simulink model "base_1fm"  (R2016b)
settings: Solver=VariableStepAuto  StartTime=0.0  StopTime=10.0  RelTol=1e-3
values from neighbouring files (symbols this model uses):
  Lb = 0.07    [base_1fm_parameters.m]
  Lf = 0.238    [base_1fm_parameters.m]
  Lu = 0.153    [base_1fm_parameters.m]
  sampleTime = 0.001    [base_1fm_parameters.m]
undefined symbols (not defined in the file or in its folder): DiscIntNeverNeededParam, RobotStruct
undefined symbols (not defined in the file): RobotStruct_FM1
libraries: simulink x27, VariousBlocksLibrary x4, FMLibrary_v2 x2, UsefulBlocksLibrary x2, simulink_extras x2, FM_Library x1
(part 2 of 3)

== system base_1fm/Robot1/DataToEtherCAT/ToActuator ==
  note: The Latched version keeps the most recent value from when the motor was on; in other words, the reason why the motor turned off.
  note: The UseActuator block can be used to enable or disable the actuator altogether.
  BusActuator : Inport
  DriveErrorIn : Inport  Port=2
  WorkspaceErrorIn : Inport  Port=3
  EnableDrive : Inport  Port=4
  DisableDrive : Inport  Port=5
  JointTorqueDes_rad : Inport  Port=6
  AppendToBus : Subsystem
  DriveEnableLogic : Subsystem
  EncodeDesiredTorque : MATLAB Function  TreatAsAtomicUnit=on  mask(EncodeDesiredTorque){transmissionRatio=ActuatorStruct.transmissionRatio, motorTorqueConstant=ActuatorStruct.motorTorqueConstant, drivePeakCurrent=ActuatorStruct.drivePeakCurrent}
      mask prompts: transmissionRatio "Transmission ratio (e.g. -8) [-]"; motorTorqueConstant "Motor torque constant [Nm/A]"; drivePeakCurrent "Motor drive peak current [A]"
      mask help:
      | Encode desired torque at the joint to torque to be produced by the motor.
      |
      | Note: due to the way the transmission is set up and the positive motor axis (clockwise is positive as seen from the motor front), there is no need to account for sign change in motor torque or encoder position.
  PreventAlgebraicLoop : Memory
  TorqueLimit_Nm : Constant  Value=ActuatorStruct.TorqueLimit_Nm
  TorqueLimiter : FM_Library/TorqueLimiter
  UseActuator : Constant  OutDataTypeStr=double
      settings: OpenFcn=|
      | b = get_param(gcb,'value');
      | if (strcmp(b,'1')),
      |   set_param (gcb,'value','0');
      | else
      |   set_param(gcb,'value','1');
      | end;
  Enable_enablecircuit : Outport
  ControlWord_drive : Outport  Port=2
  ModesOfOperation_drive : Outport  Port=3
  TargetCurrent_Drive : Outport  Port=4
  DriveErrorOut : Outport  Port=5
  DriveErrorLatched : Outport  Port=6
  ToLogger : Outport  Port=7
  wires:
  WorkspaceErrorIn/1 -> DriveEnableLogic/5(WorkspaceErrorIn)
  DriveEnableLogic/1(Enable_enablecircuit) -> Enable_enablecircuit/1
  JointTorqueDes_rad/1 -> AppendToBus/3(DesiredTorque), TorqueLimiter/2
  TorqueLimiter/1 -> DriveEnableLogic/7(TorqueGuardMax)
  TorqueLimiter/2 -> AppendToBus/4(DesiredTorqueLimited), EncodeDesiredTorque/1(JointTorque_Des_Nm)
  DriveEnableLogic/5(DriveErrorOutLatched) -> DriveErrorLatched/1
  TorqueLimit_Nm/1 -> TorqueLimiter/1
  DriveEnableLogic/3(ModesOfOperation_drive) -> ModesOfOperation_drive/1
  DriveEnableLogic/2(ControlWord_drive) -> ControlWord_drive/1
  EncodeDesiredTorque/1(MotorTorque_Des_IU) -> TargetCurrent_Drive/1
  BusActuator/1 -> DriveEnableLogic/6(BusActuators), AppendToBus/1(Bus_in)
  EnableDrive/1 -> DriveEnableLogic/1(EnableDrive)
  DisableDrive/1 -> DriveEnableLogic/2(DisableDrive)
  DriveEnableLogic/4(DriveErrorOut) -> AppendToBus/2(DriveError), PreventAlgebraicLoop/1
  DriveErrorIn/1 -> DriveEnableLogic/4(DriveErrorIn)
  PreventAlgebraicLoop/1 -> DriveErrorOut/1
  AppendToBus/1(Bus_out) -> ToLogger/1
  UseActuator/1 -> DriveEnableLogic/3(UseActuator)

== system base_1fm/Robot1/DataToEtherCAT/ToActuator1 ==
  note: The Latched version keeps the most recent value from when the motor was on; in other words, the reason why the motor turned off.
  note: The UseActuator block can be used to enable or disable the actuator altogether.
  BusActuator : Inport
  DriveErrorIn : Inport  Port=2
  WorkspaceErrorIn : Inport  Port=3
  EnableDrive : Inport  Port=4
  DisableDrive : Inport  Port=5
  JointTorqueDes_rad : Inport  Port=6
  AppendToBus : Subsystem
  DriveEnableLogic : Subsystem
  EncodeDesiredTorque : MATLAB Function  TreatAsAtomicUnit=on  mask(EncodeDesiredTorque){transmissionRatio=ActuatorStruct.transmissionRatio, motorTorqueConstant=ActuatorStruct.motorTorqueConstant, drivePeakCurrent=ActuatorStruct.drivePeakCurrent}
      mask prompts: transmissionRatio "Transmission ratio (e.g. -8) [-]"; motorTorqueConstant "Motor torque constant [Nm/A]"; drivePeakCurrent "Motor drive peak current [A]"
      mask help:
      | Encode desired torque at the joint to torque to be produced by the motor.
      |
      | Note: due to the way the transmission is set up and the positive motor axis (clockwise is positive as seen from the motor front), there is no need to account for sign change in motor torque or encoder position.
  PreventAlgebraicLoop : Memory
  TorqueLimit_Nm : Constant  Value=ActuatorStruct.TorqueLimit_Nm
  TorqueLimiter1 : Subsystem  AncestorBlock=FMLibrary_v2/Utilities/TorqueLimiter
  UseActuator : Constant  OutDataTypeStr=double
      settings: OpenFcn=|
      | b = get_param(gcb,'value');
      | if (strcmp(b,'1')),
      |   set_param (gcb,'value','0');
      | else
      |   set_param(gcb,'value','1');
      | end;
  Enable_enablecircuit : Outport
  ControlWord_drive : Outport  Port=2
  ModesOfOperation_drive : Outport  Port=3
  TargetCurrent_Drive : Outport  Port=4
  DriveErrorOut : Outport  Port=5
  DriveErrorLatched : Outport  Port=6
  ToLogger : Outport  Port=7
  wires:
  WorkspaceErrorIn/1 -> DriveEnableLogic/5(WorkspaceErrorIn)
  DriveEnableLogic/1(Enable_enablecircuit) -> Enable_enablecircuit/1
  JointTorqueDes_rad/1 -> TorqueLimiter1/2(Torque_Des_Nm), AppendToBus/3(DesiredTorque)
  TorqueLimiter1/1(Torque_GuardMax_Nm) -> DriveEnableLogic/7(TorqueGuardMax)
  TorqueLimiter1/2(Torque_Des_Limited_Nm) -> AppendToBus/4(DesiredTorqueLimited), EncodeDesiredTorque/1(JointTorque_Des_Nm)
  DriveEnableLogic/5(DriveErrorOutLatched) -> DriveErrorLatched/1
  TorqueLimit_Nm/1 -> TorqueLimiter1/1(Torque_Limit_Nm)
  DriveEnableLogic/3(ModesOfOperation_drive) -> ModesOfOperation_drive/1
  DriveEnableLogic/2(ControlWord_drive) -> ControlWord_drive/1
  EncodeDesiredTorque/1(MotorTorque_Des_IU) -> TargetCurrent_Drive/1
  BusActuator/1 -> DriveEnableLogic/6(BusActuators), AppendToBus/1(Bus_in)
  EnableDrive/1 -> DriveEnableLogic/1(EnableDrive)
  DisableDrive/1 -> DriveEnableLogic/2(DisableDrive)
  DriveEnableLogic/4(DriveErrorOut) -> AppendToBus/2(DriveError), PreventAlgebraicLoop/1
  DriveErrorIn/1 -> DriveEnableLogic/4(DriveErrorIn)
  PreventAlgebraicLoop/1 -> DriveErrorOut/1
  AppendToBus/1(Bus_out) -> ToLogger/1
  UseActuator/1 -> DriveEnableLogic/3(UseActuator)

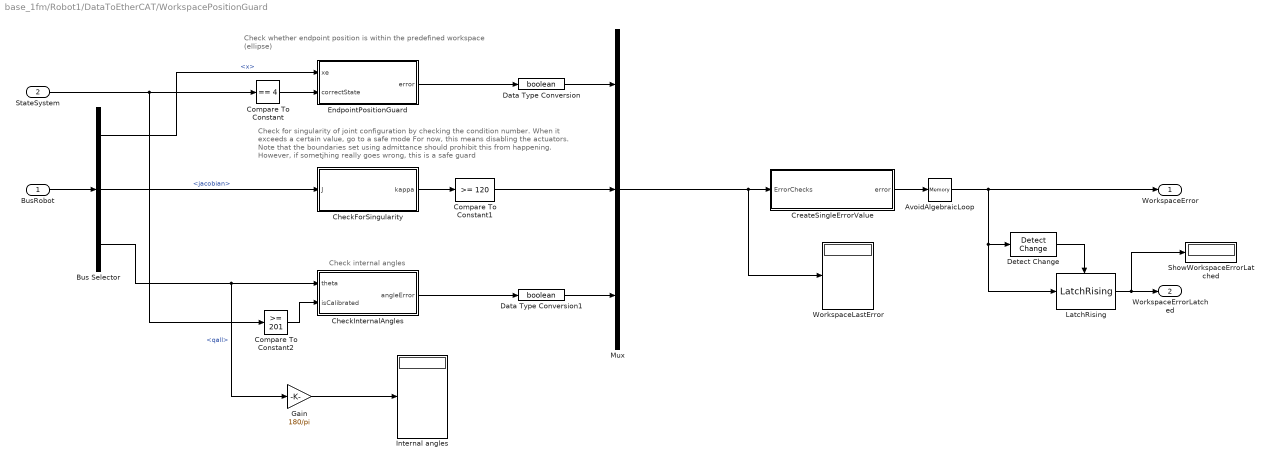
== system base_1fm/Robot1/DataToEtherCAT/WorkspacePositionGuard ==
  note: Check for singularity of joint configuration by checking
      | the condition number. When it exceeds a certain value, go to a safe mode
      | For now, this means disabling the actuators.
      | Note that the boundaries set using admittance should prohibit this from happening.
      | However, if sometjhing really goes wrong, this is a safe guard
  note: Check whether endpoint position is within the predefined workspace
      | (ellipse)
  note: Check internal angles
  BusRobot : Inport
  StateSystem : Inport  Port=2
  AvoidAlgebraicLoop : Memory
  Bus Selector : BusSelector  OutputSignals=xOpSpace.x,xOpSpace.jacobian,qJointSpace.qall
  CheckForSingularity : MATLAB Function  TreatAsAtomicUnit=on
  CheckInternalAngles : MATLAB Function  TreatAsAtomicUnit=on
  Compare To Constant : simulink/Logic and Bit Operations/Compare To Constant  relop===  const=4  OutDataTypeStr=boolean
  Compare To Constant1 : simulink/Logic and Bit Operations/Compare To Constant  relop=>=  const=120  OutDataTypeStr=boolean
  Compare To Constant2 : simulink/Logic and Bit Operations/Compare To Constant  relop=>=  const=201  OutDataTypeStr=boolean
  CreateSingleErrorValue : Subsystem
  Data Type Conversion : DataTypeConversion  OutDataTypeStr=boolean
  Data Type Conversion1 : DataTypeConversion  OutDataTypeStr=boolean
  Detect Change : simulink/Logic and Bit Operations/Detect Change  vinit=0  InputProcessing=Inherited  OutDataTypeStr=boolean
  EndpointPositionGuard : MATLAB Function  TreatAsAtomicUnit=on
  Gain : Gain  Gain=180/pi
  Internal angles : Display
  LatchRising : UsefulBlocksLibrary/LatchRising  ic=0
  Mux : Mux  Inputs=3
  ShowWorkspaceErrorLatched : Display
  WorkspaceLastError : Display
  WorkspaceError : Outport
  WorkspaceErrorLatched : Outport  Port=2
  wires:
  StateSystem/1 -> Compare To Constant/1, Compare To Constant2/1
  Bus Selector/2 -> CheckForSingularity/1(J)  "<jacobian>"
  Gain/1 -> Internal angles/1
  Compare To Constant2/1 -> CheckInternalAngles/2(isCalibrated)
  Compare To Constant/1 -> EndpointPositionGuard/2(correctState)
  AvoidAlgebraicLoop/1 -> WorkspaceError/1, LatchRising/1, Detect Change/1
  Detect Change/1 -> LatchRising/Trigger
  CreateSingleErrorValue/1(error) -> AvoidAlgebraicLoop/1
  Data Type Conversion1/1 -> Mux/3
  Data Type Conversion/1 -> Mux/1
  Compare To Constant1/1 -> Mux/2
  LatchRising/1 -> WorkspaceErrorLatched/1, ShowWorkspaceErrorLatched/1
  CheckInternalAngles/1(angleError) -> Data Type Conversion1/1
  Bus Selector/3 -> CheckInternalAngles/1(theta), Gain/1  "<qall>"
  Bus Selector/1 -> EndpointPositionGuard/1(xe)  "<x>"
  BusRobot/1 -> Bus Selector/1
  EndpointPositionGuard/1(error) -> Data Type Conversion/1
  Mux/1 -> CreateSingleErrorValue/1(ErrorChecks), WorkspaceLastError/1
  CheckForSingularity/1(kappa) -> Compare To Constant1/1

== system base_1fm/Robot1/Controller/PD + Nonlinear ID/AFFC ==
  q_ref : Inport
  qdot_ref : Inport  Port=2
  qddot_ref : Inport  Port=3
  e : Inport  Port=4
  Enable : EnablePort  StatesWhenEnabling=reset
  AFFC : MATLAB Function  TreatAsAtomicUnit=on
  Counter Free-Running : simulink/Sources/Counter Free-Running  NumBits=32  tsamp=-1
  Data Type Conversion : DataTypeConversion  OutDataTypeStr=double
  Learning factors : Constant  Value=[2e-5;1e-2;1e-3;1e-3]
  sample time : Gain  Gain=sampleTime
  p : Outport  OutputWhenDisabled=reset
  tau_affc : Outport  Port=2  OutputWhenDisabled=reset  InitialOutput=[0;0]
  wires:
  Learning factors/1 -> AFFC/6(w)
  Data Type Conversion/1 -> sample time/1
  sample time/1 -> AFFC/1(t)
  Counter Free-Running/1 -> Data Type Conversion/1
  AFFC/1(p) -> p/1
  AFFC/2(tau) -> tau_affc/1
  q_ref/1 -> AFFC/2(q)
  qdot_ref/1 -> AFFC/3(qdot)
  qddot_ref/1 -> AFFC/4(qddot)
  e/1 -> AFFC/5(e)

== system base_1fm/Robot1/DataFromEtherCAT/Calculate Arrange Joint and Op Space/forward kinematics ==
  JointPosition_rad : Inport  PortDimensions=[2 1]
  JointVelocity_rads : Inport  Port=2  PortDimensions=[2 1]
  JointAcceleration_rads2 : Inport  Port=3  PortDimensions=[2 1]
  Je : MATLAB Function  TreatAsAtomicUnit=on
  Jedot : MATLAB Function  TreatAsAtomicUnit=on
  Product : Product  Multiplication=Matrix(*)
  calculate xddot : MATLAB Function  TreatAsAtomicUnit=on
  forward kinematics : MATLAB Function  TreatAsAtomicUnit=on
  x : Outport
  xdot : Outport  Port=2
  xddot : Outport  Port=3
  J : Outport  Port=4
  Jdot : Outport  Port=5
  wires:
  JointAcceleration_rads2/1 -> calculate xddot/1(qddot)
  calculate xddot/1(xddot) -> xddot/1
  forward kinematics/1(x) -> x/1
  Product/1 -> xdot/1
  Jedot/1(Jedot) -> Jdot/1, calculate xddot/4(Jdot)
  JointVelocity_rads/1 -> Jedot/2(qdot), Product/2, calculate xddot/2(qdot)
  Je/1(Je) -> J/1, Product/1, calculate xddot/3(J)
  JointPosition_rad/1 -> Je/1(q), Jedot/1(q), forward kinematics/1(q)

== system base_1fm/Robot1/DataFromEtherCAT/FromActuator1/CalculateJointVelocity ==
  JointPosition_rad : Inport
  FOAW : MATLAB Function  TreatAsAtomicUnit=on
  encoder noise : Constant  Value=ActuatorStruct.FOAWNoiseLevel
  JointVelocity_rads : Outport
  wires:
  encoder noise/1 -> FOAW/2(noise)
  FOAW/1(xdot) -> JointVelocity_rads/1
  JointPosition_rad/1 -> FOAW/1(x)

== system base_1fm/Robot1/DataFromEtherCAT/FromActuator2/CalculateJointVelocity ==
  JointPosition_rad : Inport
  FOAW : MATLAB Function  TreatAsAtomicUnit=on
  encoder noise : Constant  Value=ActuatorStruct.FOAWNoiseLevel
  JointVelocity_rads : Outport
  wires:
  encoder noise/1 -> FOAW/2(noise)
  FOAW/1(xdot) -> JointVelocity_rads/1
  JointPosition_rad/1 -> FOAW/1(x)

== system base_1fm/Robot1/DataToEtherCAT/ToActuator/AppendToBus ==
  Bus_in : Inport
  DriveError : Inport  Port=2
  DesiredTorque : Inport  Port=3
  DesiredTorqueLimited : Inport  Port=4
  Bus Creator : BusCreator  Inputs=12
  Bus Selector2 : BusSelector  OutputSignals=OperationEnabled,StatusWord,JointPosition_rad,JointVelocity_rads,MotorEncoder_counts,MotorPosition_IncEnc_rad,JointPosition_IncEnc_rad,JointAbsoluteEncoder_counts,JointTorque_Act_Nm
  Data Type Conversion : DataTypeConversion  OutDataTypeStr=double
  Bus_out : Outport
  wires:
  Bus Selector2/9 -> Bus Creator/9  "<JointTorque_Act_Nm>"
  Bus Creator/1 -> Bus_out/1
  Bus_in/1 -> Bus Selector2/1
  DriveError/1 -> Data Type Conversion/1
  Data Type Conversion/1 -> Bus Creator/12  "DriveError"
  DesiredTorque/1 -> Bus Creator/10  "DesiredTorque_Nm"
  DesiredTorqueLimited/1 -> Bus Creator/11  "DesiredTorqueLimited_Nm"
  Bus Selector2/1 -> Bus Creator/1  "<OperationEnabled>"
  Bus Selector2/2 -> Bus Creator/2  "<StatusWord>"
  Bus Selector2/3 -> Bus Creator/3  "<JointPosition_rad>"
  Bus Selector2/4 -> Bus Creator/4  "<JointVelocity_rads>"
  Bus Selector2/5 -> Bus Creator/5  "<MotorEncoder_counts>"
  Bus Selector2/7 -> Bus Creator/7  "<JointPosition_IncEnc_rad>"
  Bus Selector2/8 -> Bus Creator/8  "<JointAbsoluteEncoder_counts>"
  Bus Selector2/6 -> Bus Creator/6  "<MotorPosition_IncEnc_rad>"

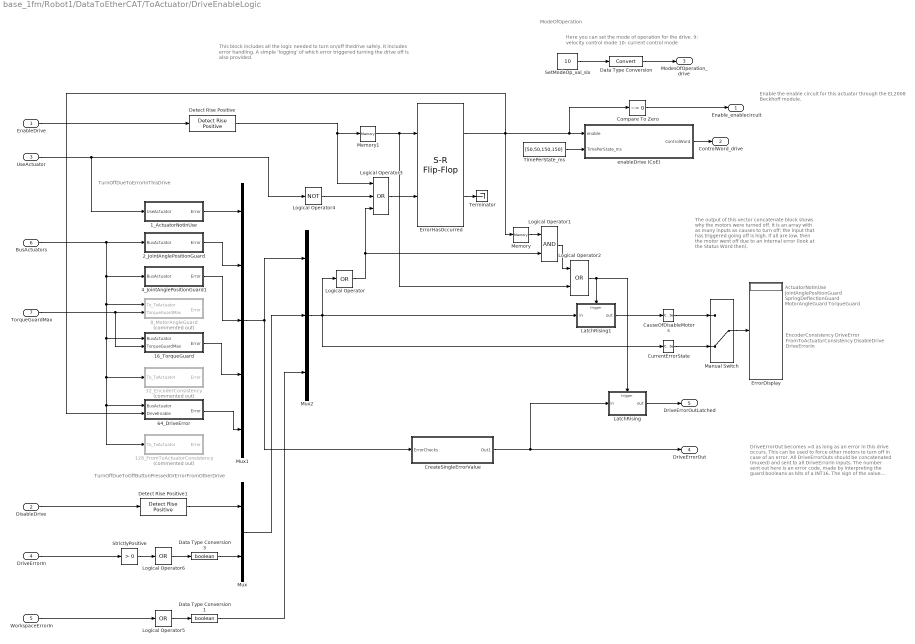
== system base_1fm/Robot1/DataToEtherCAT/ToActuator/DriveEnableLogic ==
  note: Here you can set the mode of operation for the drive.
      | 9: velocity control mode
      | 10: current control mode
  note: The output of this vector concatenate block shows why the motors were turned off. It is an array with as many inputs as causes to turn off; the input that has triggered going off is high. If all are low, then the motor went off due to an internal error (look at the Status Word then).
  note: This block includes all the logic needed to turn on/off thedrive safely. It includes error handling. A simple 'logging' of which error triggered turning the drive off is also provided.
  note: TurnOffDueToErrorInThisDrive
  note: TurnOffDueToOffButtonPressedOrErrorFromOtherDrive
  note: DriveErrorOut becomes >0 as long as an error in this drive occurs. This can be used to force other motors to turn off in case of an error.
      | All DriveErrorOuts should be concatenated (muxed)  and sent to all DriveErrorIn inputs. The number sent out here is an error code, made by interpreting the guard booleans as bits of a INT16.
      | The sign of the value indicates:
      | >=0: UseActuator=true
      | <0: UseActuator = False
  note: EncoderConsistency
      | DriveError
      | FromToActuatorConsistency
      | DisableDrive
      | DriveErrorIn
  note: ActuatorNotInUse
      | JointAnglePositionGuard
      | SpringDeflectionGuard
      | MotorAngleGuard
      | TorqueGuard
  note: ModeOfOperation
  note: Enable the enable circuit for this actuator through the EL2008
      | Beckhoff module.
  EnableDrive : Inport
  DisableDrive : Inport  Port=2
  UseActuator : Inport  Port=3
  DriveErrorIn : Inport  Port=4
  WorkspaceErrorIn : Inport  Port=5
  BusActuators : Inport  Port=6
  TorqueGuardMax : Inport  Port=7
  128_FromToActuatorConsistency : Subsystem  Commented=on
  16_TorqueGuard : Subsystem
  1_ActuatorNotInUse : Subsystem
  2_JointAnglePositionGuard : Subsystem
  32_EncoderConsistency : Subsystem  Commented=on
  4_JointAnglePositionGuard1 : Subsystem
  64_DriveError : Subsystem
  8_MotorAngleGuard : Subsystem  Commented=on
  CauseOfDisableMotors : Concatenate  NumInputs=1
  Compare To Zero : simulink/Logic and Bit Operations/Compare To Zero  relop=~=  OutDataTypeStr=boolean
  CreateSingleErrorValue : Subsystem
  CurrentErrorState : Concatenate  NumInputs=1
  Data Type Conversion : DataTypeConversion
  Data Type Conversion1 : DataTypeConversion  OutDataTypeStr=boolean
  Data Type Conversion3 : DataTypeConversion  OutDataTypeStr=boolean
  Detect Rise Positive : simulink/Logic and Bit Operations/Detect Rise Positive  vinit=0  InputProcessing=Inherited  OutDataTypeStr=boolean
  Detect Rise Positive1 : simulink/Logic and Bit Operations/Detect Rise Positive  vinit=0  InputProcessing=Inherited  OutDataTypeStr=boolean
  ErrorDisplay : Display
  ErrorHasOccurred : simulink_extras/Flip Flops/S-R Flip-Flop  initial_condition=0
  LatchRising : Subsystem  TreatAsAtomicUnit=on
  LatchRising1 : Subsystem  TreatAsAtomicUnit=on
  Logical Operator : Logic  Operator=OR  Inputs=1  AllPortsSameDT=off  OutDataTypeStr=boolean
  Logical Operator1 : Logic  AllPortsSameDT=off  OutDataTypeStr=boolean
  Logical Operator2 : Logic  Operator=OR  AllPortsSameDT=off  OutDataTypeStr=boolean
  Logical Operator3 : Logic  Operator=OR  Inputs=3  AllPortsSameDT=off  OutDataTypeStr=boolean
  Logical Operator4 : Logic  Operator=NOT  Inputs=1  AllPortsSameDT=off  OutDataTypeStr=boolean
  Logical Operator5 : Logic  Operator=OR  Inputs=1  AllPortsSameDT=off  OutDataTypeStr=boolean
  Logical Operator6 : Logic  Operator=OR  Inputs=1  AllPortsSameDT=off  OutDataTypeStr=boolean
  Manual Switch : ManualSwitch  CurrentSetting=0
  Memory : Memory
  Memory1 : Memory
  Mux : Mux  Inputs=2
  Mux1 : Mux  Inputs=5
  Mux2 : Mux  Inputs=3
  SetModeOp_val_slx : Constant  Value=10
  StrictlyPositive : simulink/Logic and Bit Operations/Compare To Zero  relop=>  OutDataTypeStr=boolean
  Terminator : Terminator
  TimePerState_ms : Constant  Value=[50,50,150,150]
  enableDrive (CoE) : MATLAB Function  TreatAsAtomicUnit=on
  Enable_enablecircuit : Outport
  ControlWord_drive : Outport  Port=2
  ModesOfOperation_drive : Outport  Port=3
  DriveErrorOut : Outport  Port=4
  DriveErrorOutLatched : Outport  Port=5
  wires:
  Data Type Conversion1/1 -> Mux2/3
  Mux1/1 -> Mux2/1, CreateSingleErrorValue/1(ErrorChecks)
  WorkspaceErrorIn/1 -> Logical Operator5/1
  Logical Operator5/1 -> Data Type Conversion1/1
  Data Type Conversion3/1 -> Mux/2
  Compare To Zero/1 -> Enable_enablecircuit/1
  16_TorqueGuard/1(Error) -> Mux1/4
  64_DriveError/1(Error) -> Mux1/5
  1_ActuatorNotInUse/1(Error) -> Mux1/1
  Logical Operator4/1 -> Logical Operator3/2
  BusActuators/1 -> 4_JointAnglePositionGuard1/1(BusActuator), 32_EncoderConsistency/1(To_ToActuator), 64_DriveError/1(BusActuator), 128_FromToActuatorConsistency/1(To_ToActuator), 16_TorqueGuard/1(BusActuator), 8_MotorAngleGuard/1(To_ToActuator), 2_JointAnglePositionGuard/1(BusActuator)
  Mux/1 -> Mux2/2
  Logical Operator6/1 -> Data Type Conversion3/1
  DriveErrorIn/1 -> StrictlyPositive/1
  UseActuator/1 -> Logical Operator4/1, 1_ActuatorNotInUse/1(UseActuator)
  TimePerState_ms/1 -> enableDrive (CoE)/2(TimePerState_ms)
  Detect Rise Positive/1 -> Memory1/1, Logical Operator3/1
  Logical Operator3/1 -> ErrorHasOccurred/2
  Manual Switch/1 -> ErrorDisplay/1
  Logical Operator1/1 -> Logical Operator2/1
  CurrentErrorState/1 -> Manual Switch/2
  Logical Operator2/1 -> LatchRising/Trigger, LatchRising1/Trigger
  Memory/1 -> Logical Operator1/1
  Memory1/1 -> ErrorHasOccurred/1, Logical Operator2/2
  CauseOfDisableMotors/1 -> Manual Switch/1
  Data Type Conversion/1 -> ModesOfOperation_drive/1
  ErrorHasOccurred/2 -> Terminator/1
  DisableDrive/1 -> Detect Rise Positive1/1
  Detect Rise Positive1/1 -> Mux/1
  Mux2/1 -> LatchRising1/1(in), CurrentErrorState/1, Logical Operator/1
  ErrorHasOccurred/1 -> enableDrive (CoE)/1(enable), Compare To Zero/1, 64_DriveError/2(DriveEnable), Memory/1
  enableDrive (CoE)/1(ControlWord) -> ControlWord_drive/1
  EnableDrive/1 -> Detect Rise Positive/1
  SetModeOp_val_slx/1 -> Data Type Conversion/1
  Logical Operator/1 -> Logical Operator1/2, Logical Operator3/3
  LatchRising1/1(out) -> CauseOfDisableMotors/1
  TorqueGuardMax/1 -> 8_MotorAngleGuard/2(TorqueGuardMax), 16_TorqueGuard/2(TorqueGuardMax)
  StrictlyPositive/1 -> Logical Operator6/1
  CreateSingleErrorValue/1(Out1) -> LatchRising/1(in), DriveErrorOut/1
  LatchRising/1(out) -> DriveErrorOutLatched/1
  4_JointAnglePositionGuard1/1(Error) -> Mux1/3
  2_JointAnglePositionGuard/1(Error) -> Mux1/2

== system base_1fm/Robot1/DataToEtherCAT/ToActuator1/AppendToBus ==
  Bus_in : Inport
  DriveError : Inport  Port=2
  DesiredTorque : Inport  Port=3
  DesiredTorqueLimited : Inport  Port=4
  Bus Creator : BusCreator  Inputs=12
  Bus Selector2 : BusSelector  OutputSignals=OperationEnabled,StatusWord,JointPosition_rad,JointVelocity_rads,MotorEncoder_counts,MotorPosition_IncEnc_rad,JointPosition_IncEnc_rad,JointAbsoluteEncoder_counts,JointTorque_Act_Nm
  Data Type Conversion : DataTypeConversion  OutDataTypeStr=double
  Bus_out : Outport
  wires:
  Bus Selector2/9 -> Bus Creator/9  "<JointTorque_Act_Nm>"
  Bus Creator/1 -> Bus_out/1
  Bus_in/1 -> Bus Selector2/1
  DriveError/1 -> Data Type Conversion/1
  Data Type Conversion/1 -> Bus Creator/12  "DriveError"
  DesiredTorque/1 -> Bus Creator/10  "DesiredTorque_Nm"
  DesiredTorqueLimited/1 -> Bus Creator/11  "DesiredTorqueLimited_Nm"
  Bus Selector2/1 -> Bus Creator/1  "<OperationEnabled>"
  Bus Selector2/2 -> Bus Creator/2  "<StatusWord>"
  Bus Selector2/3 -> Bus Creator/3  "<JointPosition_rad>"
  Bus Selector2/4 -> Bus Creator/4  "<JointVelocity_rads>"
  Bus Selector2/5 -> Bus Creator/5  "<MotorEncoder_counts>"
  Bus Selector2/7 -> Bus Creator/7  "<JointPosition_IncEnc_rad>"
  Bus Selector2/8 -> Bus Creator/8  "<JointAbsoluteEncoder_counts>"
  Bus Selector2/6 -> Bus Creator/6  "<MotorPosition_IncEnc_rad>"

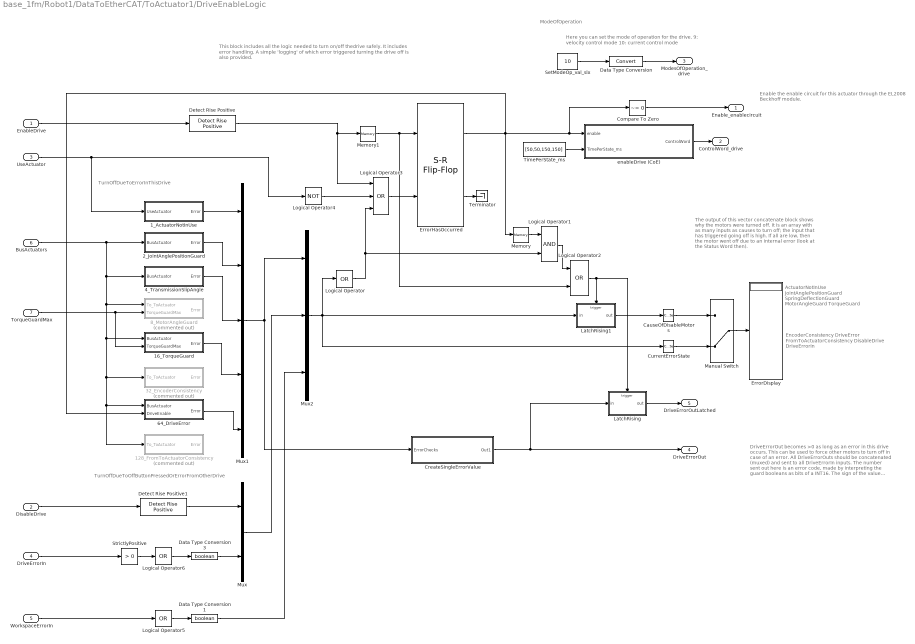
== system base_1fm/Robot1/DataToEtherCAT/ToActuator1/DriveEnableLogic ==
  note: Here you can set the mode of operation for the drive.
      | 9: velocity control mode
      | 10: current control mode
  note: The output of this vector concatenate block shows why the motors were turned off. It is an array with as many inputs as causes to turn off; the input that has triggered going off is high. If all are low, then the motor went off due to an internal error (look at the Status Word then).
  note: This block includes all the logic needed to turn on/off thedrive safely. It includes error handling. A simple 'logging' of which error triggered turning the drive off is also provided.
  note: TurnOffDueToErrorInThisDrive
  note: TurnOffDueToOffButtonPressedOrErrorFromOtherDrive
  note: DriveErrorOut becomes >0 as long as an error in this drive occurs. This can be used to force other motors to turn off in case of an error.
      | All DriveErrorOuts should be concatenated (muxed)  and sent to all DriveErrorIn inputs. The number sent out here is an error code, made by interpreting the guard booleans as bits of a INT16.
      | The sign of the value indicates:
      | >=0: UseActuator=true
      | <0: UseActuator = False
  note: EncoderConsistency
      | DriveError
      | FromToActuatorConsistency
      | DisableDrive
      | DriveErrorIn
  note: ActuatorNotInUse
      | JointAnglePositionGuard
      | SpringDeflectionGuard
      | MotorAngleGuard
      | TorqueGuard
  note: ModeOfOperation
  note: Enable the enable circuit for this actuator through the EL2008
      | Beckhoff module.
  EnableDrive : Inport
  DisableDrive : Inport  Port=2
  UseActuator : Inport  Port=3
  DriveErrorIn : Inport  Port=4
  WorkspaceErrorIn : Inport  Port=5
  BusActuators : Inport  Port=6
  TorqueGuardMax : Inport  Port=7
  128_FromToActuatorConsistency : Subsystem  Commented=on
  16_TorqueGuard : Subsystem
  1_ActuatorNotInUse : Subsystem
  2_JointAnglePositionGuard : Subsystem
  32_EncoderConsistency : Subsystem  Commented=on
  4_TransmissionSlipAngle : Subsystem
  64_DriveError : Subsystem
  8_MotorAngleGuard : Subsystem  Commented=on
  CauseOfDisableMotors : Concatenate  NumInputs=1
  Compare To Zero : simulink/Logic and Bit Operations/Compare To Zero  relop=~=  OutDataTypeStr=boolean
  CreateSingleErrorValue : Subsystem
  CurrentErrorState : Concatenate  NumInputs=1
  Data Type Conversion : DataTypeConversion
  Data Type Conversion1 : DataTypeConversion  OutDataTypeStr=boolean
  Data Type Conversion3 : DataTypeConversion  OutDataTypeStr=boolean
  Detect Rise Positive : simulink/Logic and Bit Operations/Detect Rise Positive  vinit=0  InputProcessing=Inherited  OutDataTypeStr=boolean
  Detect Rise Positive1 : simulink/Logic and Bit Operations/Detect Rise Positive  vinit=0  InputProcessing=Inherited  OutDataTypeStr=boolean
  ErrorDisplay : Display
  ErrorHasOccurred : simulink_extras/Flip Flops/S-R Flip-Flop  initial_condition=0
  LatchRising : Subsystem  TreatAsAtomicUnit=on
  LatchRising1 : Subsystem  TreatAsAtomicUnit=on
  Logical Operator : Logic  Operator=OR  Inputs=1  AllPortsSameDT=off  OutDataTypeStr=boolean
  Logical Operator1 : Logic  AllPortsSameDT=off  OutDataTypeStr=boolean
  Logical Operator2 : Logic  Operator=OR  AllPortsSameDT=off  OutDataTypeStr=boolean
  Logical Operator3 : Logic  Operator=OR  Inputs=3  AllPortsSameDT=off  OutDataTypeStr=boolean
  Logical Operator4 : Logic  Operator=NOT  Inputs=1  AllPortsSameDT=off  OutDataTypeStr=boolean
  Logical Operator5 : Logic  Operator=OR  Inputs=1  AllPortsSameDT=off  OutDataTypeStr=boolean
  Logical Operator6 : Logic  Operator=OR  Inputs=1  AllPortsSameDT=off  OutDataTypeStr=boolean
  Manual Switch : ManualSwitch  CurrentSetting=0
  Memory : Memory
  Memory1 : Memory
  Mux : Mux  Inputs=2
  Mux1 : Mux  Inputs=5
  Mux2 : Mux  Inputs=3
  SetModeOp_val_slx : Constant  Value=10
  StrictlyPositive : simulink/Logic and Bit Operations/Compare To Zero  relop=>  OutDataTypeStr=boolean
  Terminator : Terminator
  TimePerState_ms : Constant  Value=[50,50,150,150]
  enableDrive (CoE) : MATLAB Function  TreatAsAtomicUnit=on
  Enable_enablecircuit : Outport
  ControlWord_drive : Outport  Port=2
  ModesOfOperation_drive : Outport  Port=3
  DriveErrorOut : Outport  Port=4
  DriveErrorOutLatched : Outport  Port=5
  wires:
  Data Type Conversion1/1 -> Mux2/3
  Mux1/1 -> Mux2/1, CreateSingleErrorValue/1(ErrorChecks)
  WorkspaceErrorIn/1 -> Logical Operator5/1
  Logical Operator5/1 -> Data Type Conversion1/1
  Data Type Conversion3/1 -> Mux/2
  Compare To Zero/1 -> Enable_enablecircuit/1
  16_TorqueGuard/1(Error) -> Mux1/4
  64_DriveError/1(Error) -> Mux1/5
  1_ActuatorNotInUse/1(Error) -> Mux1/1
  Logical Operator4/1 -> Logical Operator3/2
  BusActuators/1 -> 4_TransmissionSlipAngle/1(BusActuator), 32_EncoderConsistency/1(To_ToActuator), 64_DriveError/1(BusActuator), 128_FromToActuatorConsistency/1(To_ToActuator), 16_TorqueGuard/1(BusActuator), 8_MotorAngleGuard/1(To_ToActuator), 2_JointAnglePositionGuard/1(BusActuator)
  Mux/1 -> Mux2/2
  Logical Operator6/1 -> Data Type Conversion3/1
  DriveErrorIn/1 -> StrictlyPositive/1
  UseActuator/1 -> Logical Operator4/1, 1_ActuatorNotInUse/1(UseActuator)
  TimePerState_ms/1 -> enableDrive (CoE)/2(TimePerState_ms)
  Detect Rise Positive/1 -> Memory1/1, Logical Operator3/1
  Logical Operator3/1 -> ErrorHasOccurred/2
  Manual Switch/1 -> ErrorDisplay/1
  Logical Operator1/1 -> Logical Operator2/1
  CurrentErrorState/1 -> Manual Switch/2
  Logical Operator2/1 -> LatchRising/Trigger, LatchRising1/Trigger
  Memory/1 -> Logical Operator1/1
  Memory1/1 -> ErrorHasOccurred/1, Logical Operator2/2
  CauseOfDisableMotors/1 -> Manual Switch/1
  Data Type Conversion/1 -> ModesOfOperation_drive/1
  ErrorHasOccurred/2 -> Terminator/1
  DisableDrive/1 -> Detect Rise Positive1/1
  Detect Rise Positive1/1 -> Mux/1
  Mux2/1 -> LatchRising1/1(in), CurrentErrorState/1, Logical Operator/1
  ErrorHasOccurred/1 -> enableDrive (CoE)/1(enable), Compare To Zero/1, 64_DriveError/2(DriveEnable), Memory/1
  enableDrive (CoE)/1(ControlWord) -> ControlWord_drive/1
  EnableDrive/1 -> Detect Rise Positive/1
  SetModeOp_val_slx/1 -> Data Type Conversion/1
  Logical Operator/1 -> Logical Operator1/2, Logical Operator3/3
  LatchRising1/1(out) -> CauseOfDisableMotors/1
  TorqueGuardMax/1 -> 8_MotorAngleGuard/2(TorqueGuardMax), 16_TorqueGuard/2(TorqueGuardMax)
  StrictlyPositive/1 -> Logical Operator6/1
  CreateSingleErrorValue/1(Out1) -> LatchRising/1(in), DriveErrorOut/1
  LatchRising/1(out) -> DriveErrorOutLatched/1
  4_TransmissionSlipAngle/1(Error) -> Mux1/3
  2_JointAnglePositionGuard/1(Error) -> Mux1/2

== system base_1fm/Robot1/DataToEtherCAT/ToActuator1/TorqueLimiter1 ==
  note: This block limits the Desird Torque to an interval [-TorqueLimit, +TorqueLimit]. It also sets TorqueGuardMax_Nm to 0.5 Nm more than the TorqueLimit. This is used in the DriveEnableLogic block to completely shut down the motor (and with that, all other motors) if the limit is severly (by 0.5 Nm) exceeded.
      |
      | Note that the actuators are rated to a maximum of 4 Nm, so if the user puts a TorqueLimit of higher than 4 Nm in, this block will still limit it to 4 Nm.
  Torque_Limit_Nm : Inport
  Torque_Des_Nm : Inport  Port=2
  AbsoluteMaximumTorque_Nm : Constant  Value=ActuatorStruct.AbsoluteMaximumTorque_Nm
  Bias : Bias  Bias=0.5
  MinMax : MinMax  Inputs=2
  Saturation Dynamic : simulink/Discontinuities/Saturation Dynamic  OutMin=[]  OutMax=[]  OutDataTypeStr=Inherit: Same as second input  OutDataType=fixdt(1, 16)  OutScaling=2^-10  DoSatur=off
  Unary Minus : UnaryMinus
  Torque_GuardMax_Nm : Outport
  Torque_Des_Limited_Nm : Outport  Port=2
  wires:
  Torque_Limit_Nm/1 -> MinMax/1
  AbsoluteMaximumTorque_Nm/1 -> MinMax/2
  MinMax/1 -> Bias/1, Unary Minus/1, Saturation Dynamic/1
  Unary Minus/1 -> Saturation Dynamic/3
  Saturation Dynamic/1 -> Torque_Des_Limited_Nm/1
  Torque_Des_Nm/1 -> Saturation Dynamic/2
  Bias/1 -> Torque_GuardMax_Nm/1

== system base_1fm/Robot1/DataToEtherCAT/WorkspacePositionGuard/CreateSingleErrorValue ==
  ErrorChecks : Inport
  Data Type Conversion1 : DataTypeConversion  OutDataTypeStr=double
  Data Type Conversion2 : DataTypeConversion  OutDataTypeStr=int32
  MATLAB Function : MATLAB Function  TreatAsAtomicUnit=on
  error : Outport
  wires:
  Data Type Conversion2/1 -> error/1
  ErrorChecks/1 -> Data Type Conversion1/1
  Data Type Conversion1/1 -> MATLAB Function/1(errors)
  MATLAB Function/1(out) -> Data Type Conversion2/1

== system base_1fm/Robot1/DataToEtherCAT/ToActuator/DriveEnableLogic/128_FromToActuatorConsistency ==
  note: This block checks whether the FromActuator and ToActuator blocks use the same ActuatorStruct. If not, you've done something wrong. It does this by checking if the JointEncoderOffsets are identical.
  To_ToActuator : Inport
  Bus Selector : BusSelector  OutputSignals=JointEncoderOffset
  Constant : Constant  Value=ActuatorStruct.JointEncoderOffset
  Relational Operator : RelationalOperator  Operator=~=  OutDataTypeStr=boolean  RndMeth=Nearest
  Error : Outport
  wires:
  Constant/1 -> Relational Operator/2
  Bus Selector/1 -> Relational Operator/1  "<JointEncoderOffset>"
  Relational Operator/1 -> Error/1
  To_ToActuator/1 -> Bus Selector/1

== system base_1fm/Robot1/DataToEtherCAT/ToActuator/DriveEnableLogic/16_TorqueGuard ==
  BusActuator : Inport
  TorqueGuardMax : Inport  Port=2
  Abs : Abs
  Bus Selector : BusSelector  OutputSignals=JointTorque_Act_Nm
  Relational Operator : RelationalOperator  Operator=>  OutDataTypeStr=boolean  RndMeth=Nearest
  Error : Outport  PortDimensions=1
  wires:
  Relational Operator/1 -> Error/1
  Abs/1 -> Relational Operator/1
  BusActuator/1 -> Bus Selector/1
  Bus Selector/1 -> Abs/1  "<JointTorque_Act_Nm>"
  TorqueGuardMax/1 -> Relational Operator/2

== system base_1fm/Robot1/DataToEtherCAT/ToActuator/DriveEnableLogic/1_ActuatorNotInUse ==
  note: When UseActuator = 0, this block outputs 1. Later in the chain, the ErrorValue is then negated, resulting in -1 if there are no other errors. Note, thus, that this output does not really indicate an error; more a status.
  UseActuator : Inport
  Logical Operator1 : Logic  Operator=NOT  AllPortsSameDT=off  OutDataTypeStr=boolean
  Error : Outport  PortDimensions=1
  wires:
  UseActuator/1 -> Logical Operator1/1
  Logical Operator1/1 -> Error/1

== system base_1fm/Robot1/DataToEtherCAT/ToActuator/DriveEnableLogic/2_JointAnglePositionGuard ==
  note: This block makes sure that the motors are turned off (and cannot go on) when the joint is outside its normal range.
  BusActuator : Inport
  Bus Selector : BusSelector  OutputSignals=JointPosition_rad
  Logical Operator : Logic  Operator=OR  AllPortsSameDT=off  OutDataTypeStr=boolean
  Maximum : Constant  Value=ActuatorStruct.JointPositionGuardMax
  Minimum : Constant  Value=ActuatorStruct.JointPositionGuardMin
  Relational Operator : RelationalOperator  Operator=<=  OutDataTypeStr=boolean  RndMeth=Nearest
  Relational Operator1 : RelationalOperator  OutDataTypeStr=boolean  RndMeth=Nearest
  Error : Outport
  wires:
  Bus Selector/1 -> Relational Operator/1, Relational Operator1/1  "<JointPosition_rad>"
  Maximum/1 -> Relational Operator1/2
  Minimum/1 -> Relational Operator/2
  Logical Operator/1 -> Error/1
  Relational Operator1/1 -> Logical Operator/2
  Relational Operator/1 -> Logical Operator/1
  BusActuator/1 -> Bus Selector/1

== system base_1fm/Robot1/DataToEtherCAT/ToActuator/DriveEnableLogic/32_EncoderConsistency ==
  note: This block checks whether the three encoders are consistent. Ideally, the sum (with jointAngle negated) should be exactly zero at all times (also when forces are exerted). We allow some room around it however.
  To_ToActuator : Inport
  Abs : Abs
  Add : Sum  Inputs=+-
  Bus Selector : BusSelector  OutputSignals=JointPosition_IncEnc_rad,JointPosition_AbsEnc_rad
  Compare To Constant : simulink/Logic and Bit Operations/Compare To Constant  relop=<=  const=3.0  OutDataTypeStr=boolean
  EncoderInConsistency_rad : Concatenate  NumInputs=1
  Error : Outport
  wires:
  EncoderInConsistency_rad/1 -> Abs/1
  Add/1 -> EncoderInConsistency_rad/1
  Bus Selector/2 -> Add/2  "<JointPosition_AbsEnc_rad>"
  Abs/1 -> Compare To Constant/1
  Compare To Constant/1 -> Error/1
  To_ToActuator/1 -> Bus Selector/1
  Bus Selector/1 -> Add/1  "<JointPosition_IncEnc_rad>"

== system base_1fm/Robot1/DataToEtherCAT/ToActuator/DriveEnableLogic/4_JointAnglePositionGuard1 ==
  note: This block makes sure that the motors are turned off when the transmission slips.
  BusActuator : Inport
  Bus Selector : BusSelector  OutputSignals=JointPosition_rad,JointPosition_IncEnc_rad
  Minimum : Constant  Value=ActuatorStruct.TransmissionSlipAngleGuardMax
  Relational Operator1 : RelationalOperator  OutDataTypeStr=boolean  RndMeth=Nearest
  Subtract : Sum  Inputs=+-
  Error : Outport
  wires:
  Bus Selector/1 -> Subtract/1  "<JointPosition_rad>"
  Relational Operator1/1 -> Error/1
  BusActuator/1 -> Bus Selector/1
  Minimum/1 -> Relational Operator1/2
  Bus Selector/2 -> Subtract/2  "<JointPosition_IncEnc_rad>"
  Subtract/1 -> Relational Operator1/1

== system base_1fm/Robot1/DataToEtherCAT/ToActuator/DriveEnableLogic/64_DriveError ==
  note: This block checks whether the drive went off by itself. Reasons why this could happen are: undervoltage of the motor power supply, short-circuit detection triggered, I2t error etc.
      | The first few seconds that the drive should be on (i.e., DriveEnable = True), the drive is in the process of turning on, and will not be really on. In order to avoid direct turn-off due to this, we disable this error the first few seconds.
  note: This memory block is to avoid an
      | algebraic loop
  note: This memory block is to avoid that this error 'turns on' when another error is triggered.
  BusActuator : Inport
  DriveEnable : Inport  Port=2
  Bus Selector : BusSelector  OutputSignals=OperationEnabled
  CountHowLongEnableWasTrue : MATLAB Function  TreatAsAtomicUnit=on
  InhibitTime_s : Constant  Value=2.0
  Logical Operator : Logic  AllPortsSameDT=off  OutDataTypeStr=boolean
  Logical Operator2 : Logic  Operator=NOT  AllPortsSameDT=off  OutDataTypeStr=boolean
  Memory : Memory
  Memory1 : Memory
  Relational Operator : RelationalOperator  OutDataTypeStr=boolean  RndMeth=Nearest
  ToSeconds : Gain  Gain=sampleTime
  Error : Outport  PortDimensions=1
  wires:
  Logical Operator2/1 -> Logical Operator/2
  Memory1/1 -> Bus Selector/1
  Memory/1 -> CountHowLongEnableWasTrue/1(u)
  InhibitTime_s/1 -> Relational Operator/2
  Relational Operator/1 -> Logical Operator/1
  ToSeconds/1 -> Relational Operator/1
  CountHowLongEnableWasTrue/1(y) -> ToSeconds/1
  DriveEnable/1 -> Memory/1
  Bus Selector/1 -> Logical Operator2/1  "<OperationEnabled>"
  BusActuator/1 -> Memory1/1
  Logical Operator/1 -> Error/1

== system base_1fm/Robot1/DataToEtherCAT/ToActuator/DriveEnableLogic/8_MotorAngleGuard ==
  note: This block checks whether the motor encoder gives sensible data, i.e., if the motor angle is within the expected range. The expected range is the full stroke of the output shaft plus the maximum spring deflection, transformed to motor angle space.
  To_ToActuator : Inport
  TorqueGuardMax : Inport  Port=2
  Add : Sum  Inputs=+-
  Add1 : Sum
  Bus Selector : BusSelector  OutputSignals=MotorPosition_IncEnc_rad
  Divide : Product  Inputs=*/
  Logical Operator : Logic  Operator=OR  AllPortsSameDT=off  OutDataTypeStr=boolean
  Maximum : Constant  Value=ActuatorStruct.JointAnglePositionGuardMax_rad
  Minimum : Constant  Value=ActuatorStruct.JointAnglePositionGuardMin_rad
  Relational Operator1 : RelationalOperator  Operator=<=  OutDataTypeStr=boolean  RndMeth=Nearest
  Relational Operator2 : RelationalOperator  OutDataTypeStr=boolean  RndMeth=Nearest
  SpringStiffness : Constant  Value=ActuatorStruct.SpringStiffness_Nm_rad
  TransformToMotorSpace : Gain  Gain=ActuatorStruct.gearboxRatio
  TransformToMotorSpace1 : Gain  Gain=ActuatorStruct.gearboxRatio
  Error : Outport
  wires:
  Minimum/1 -> Add/1
  Divide/1 -> Add1/2, Add/2  "MaximumSpringDeflection_rad"
  Maximum/1 -> Add1/1
  SpringStiffness/1 -> Divide/2
  TorqueGuardMax/1 -> Divide/1
  TransformToMotorSpace/1 -> Relational Operator2/2
  Add/1 -> TransformToMotorSpace1/1
  Add1/1 -> TransformToMotorSpace/1
  TransformToMotorSpace1/1 -> Relational Operator1/2
  Logical Operator/1 -> Error/1
  Relational Operator2/1 -> Logical Operator/2
  Relational Operator1/1 -> Logical Operator/1
  Bus Selector/1 -> Relational Operator1/1, Relational Operator2/1  "<MotorPosition_IncEnc_rad>"
  To_ToActuator/1 -> Bus Selector/1

== system base_1fm/Robot1/DataToEtherCAT/ToActuator/DriveEnableLogic/CreateSingleErrorValue ==
  ErrorChecks : Inport
  Data Type Conversion1 : DataTypeConversion  OutDataTypeStr=double
  Data Type Conversion2 : DataTypeConversion  OutDataTypeStr=int32
  MATLAB Function : MATLAB Function  TreatAsAtomicUnit=on
  Select_NotUseActuator : Selector  InputPortWidth=3  IndexOptions=Index vector (dialog)  Indices=1  OutputSizes=1
  Switch : Switch  Criteria=u2 ~= 0
  Unary Minus : UnaryMinus
  Out1 : Outport
  wires:
  Unary Minus/1 -> Switch/1
  Switch/1 -> Out1/1
  ErrorChecks/1 -> Data Type Conversion1/1
  Select_NotUseActuator/1 -> Switch/2
  Data Type Conversion1/1 -> Select_NotUseActuator/1, MATLAB Function/1(errors)
  MATLAB Function/1(out) -> Data Type Conversion2/1
  Data Type Conversion2/1 -> Unary Minus/1, Switch/3

== system base_1fm/Robot1/DataToEtherCAT/ToActuator/DriveEnableLogic/LatchRising ==
  in : Inport
  Trigger : TriggerPort  VariantControl=Variant  PortDimensions=1
  out : Outport
  wires:
  in/1 -> out/1

== system base_1fm/Robot1/DataToEtherCAT/ToActuator/DriveEnableLogic/LatchRising1 ==
  in : Inport
  Trigger : TriggerPort  VariantControl=Variant  PortDimensions=1
  out : Outport
  wires:
  in/1 -> out/1

== system base_1fm/Robot1/DataToEtherCAT/ToActuator1/DriveEnableLogic/128_FromToActuatorConsistency ==
  note: This block checks whether the FromActuator and ToActuator blocks use the same ActuatorStruct. If not, you've done something wrong. It does this by checking if the JointEncoderOffsets are identical.
  To_ToActuator : Inport
  Bus Selector : BusSelector  OutputSignals=JointEncoderOffset
  Constant : Constant  Value=ActuatorStruct.JointEncoderOffset
  Relational Operator : RelationalOperator  Operator=~=  OutDataTypeStr=boolean  RndMeth=Nearest
  Error : Outport
  wires:
  Constant/1 -> Relational Operator/2
  Bus Selector/1 -> Relational Operator/1  "<JointEncoderOffset>"
  Relational Operator/1 -> Error/1
  To_ToActuator/1 -> Bus Selector/1

== system base_1fm/Robot1/DataToEtherCAT/ToActuator1/DriveEnableLogic/16_TorqueGuard ==
  BusActuator : Inport
  TorqueGuardMax : Inport  Port=2
  Abs : Abs
  Bus Selector : BusSelector  OutputSignals=JointTorque_Act_Nm
  Relational Operator : RelationalOperator  Operator=>  OutDataTypeStr=boolean  RndMeth=Nearest
  Error : Outport  PortDimensions=1
  wires:
  Relational Operator/1 -> Error/1
  Abs/1 -> Relational Operator/1
  BusActuator/1 -> Bus Selector/1
  Bus Selector/1 -> Abs/1  "<JointTorque_Act_Nm>"
  TorqueGuardMax/1 -> Relational Operator/2

== system base_1fm/Robot1/DataToEtherCAT/ToActuator1/DriveEnableLogic/1_ActuatorNotInUse ==
  note: When UseActuator = 0, this block outputs 1. Later in the chain, the ErrorValue is then negated, resulting in -1 if there are no other errors. Note, thus, that this output does not really indicate an error; more a status.
  UseActuator : Inport
  Logical Operator1 : Logic  Operator=NOT  AllPortsSameDT=off  OutDataTypeStr=boolean
  Error : Outport  PortDimensions=1
  wires:
  UseActuator/1 -> Logical Operator1/1
  Logical Operator1/1 -> Error/1

== system base_1fm/Robot1/DataToEtherCAT/ToActuator1/DriveEnableLogic/2_JointAnglePositionGuard ==
  note: This block makes sure that the motors are turned off (and cannot go on) when the joint is outside its normal range.
  BusActuator : Inport
  Bus Selector : BusSelector  OutputSignals=JointPosition_rad
  Logical Operator : Logic  Operator=OR  AllPortsSameDT=off  OutDataTypeStr=boolean
  Maximum : Constant  Value=ActuatorStruct.JointPositionGuardMax
  Minimum : Constant  Value=ActuatorStruct.JointPositionGuardMin
  Relational Operator : RelationalOperator  Operator=<=  OutDataTypeStr=boolean  RndMeth=Nearest
  Relational Operator1 : RelationalOperator  OutDataTypeStr=boolean  RndMeth=Nearest
  Error : Outport
  wires:
  Bus Selector/1 -> Relational Operator/1, Relational Operator1/1  "<JointPosition_rad>"
  Maximum/1 -> Relational Operator1/2
  Minimum/1 -> Relational Operator/2
  Logical Operator/1 -> Error/1
  Relational Operator1/1 -> Logical Operator/2
  Relational Operator/1 -> Logical Operator/1
  BusActuator/1 -> Bus Selector/1

== system base_1fm/Robot1/DataToEtherCAT/ToActuator1/DriveEnableLogic/32_EncoderConsistency ==
  note: This block checks whether the three encoders are consistent. Ideally, the sum (with jointAngle negated) should be exactly zero at all times (also when forces are exerted). We allow some room around it however.
  To_ToActuator : Inport
  Abs : Abs
  Add : Sum  Inputs=+-
  Bus Selector : BusSelector  OutputSignals=JointPosition_IncEnc_rad,JointPosition_AbsEnc_rad
  Compare To Constant : simulink/Logic and Bit Operations/Compare To Constant  relop=<=  const=3.0  OutDataTypeStr=boolean
  EncoderInConsistency_rad : Concatenate  NumInputs=1
  Error : Outport
  wires:
  EncoderInConsistency_rad/1 -> Abs/1
  Add/1 -> EncoderInConsistency_rad/1
  Bus Selector/2 -> Add/2  "<JointPosition_AbsEnc_rad>"
  Abs/1 -> Compare To Constant/1
  Compare To Constant/1 -> Error/1
  To_ToActuator/1 -> Bus Selector/1
  Bus Selector/1 -> Add/1  "<JointPosition_IncEnc_rad>"

== system base_1fm/Robot1/DataToEtherCAT/ToActuator1/DriveEnableLogic/4_TransmissionSlipAngle ==
  note: This block makes sure that the motors are turned off when the transmission slips.
  BusActuator : Inport
  Bus Selector : BusSelector  OutputSignals=JointPosition_rad,JointPosition_IncEnc_rad
  Minimum : Constant  Value=ActuatorStruct.TransmissionSlipAngleGuardMax
  Relational Operator1 : RelationalOperator  OutDataTypeStr=boolean  RndMeth=Nearest
  Subtract : Sum  Inputs=+-
  Error : Outport
  wires:
  Bus Selector/1 -> Subtract/1  "<JointPosition_rad>"
  Relational Operator1/1 -> Error/1
  BusActuator/1 -> Bus Selector/1
  Minimum/1 -> Relational Operator1/2
  Bus Selector/2 -> Subtract/2  "<JointPosition_IncEnc_rad>"
  Subtract/1 -> Relational Operator1/1

== system base_1fm/Robot1/DataToEtherCAT/ToActuator1/DriveEnableLogic/64_DriveError ==
  note: This block checks whether the drive went off by itself. Reasons why this could happen are: undervoltage of the motor power supply, short-circuit detection triggered, I2t error etc.
      | The first few seconds that the drive should be on (i.e., DriveEnable = True), the drive is in the process of turning on, and will not be really on. In order to avoid direct turn-off due to this, we disable this error the first few seconds.
  note: This memory block is to avoid an
      | algebraic loop
  note: This memory block is to avoid that this error 'turns on' when another error is triggered.
  BusActuator : Inport
  DriveEnable : Inport  Port=2
  Bus Selector : BusSelector  OutputSignals=OperationEnabled
  CountHowLongEnableWasTrue : MATLAB Function  TreatAsAtomicUnit=on
  InhibitTime_s : Constant  Value=2.0
  Logical Operator : Logic  AllPortsSameDT=off  OutDataTypeStr=boolean
  Logical Operator2 : Logic  Operator=NOT  AllPortsSameDT=off  OutDataTypeStr=boolean
  Memory : Memory
  Memory1 : Memory
  Relational Operator : RelationalOperator  OutDataTypeStr=boolean  RndMeth=Nearest
  ToSeconds : Gain  Gain=sampleTime
  Error : Outport  PortDimensions=1
  wires:
  Logical Operator2/1 -> Logical Operator/2
  Memory1/1 -> Bus Selector/1
  Memory/1 -> CountHowLongEnableWasTrue/1(u)
  InhibitTime_s/1 -> Relational Operator/2
  Relational Operator/1 -> Logical Operator/1
  ToSeconds/1 -> Relational Operator/1
  CountHowLongEnableWasTrue/1(y) -> ToSeconds/1
  DriveEnable/1 -> Memory/1
  Bus Selector/1 -> Logical Operator2/1  "<OperationEnabled>"
  BusActuator/1 -> Memory1/1
  Logical Operator/1 -> Error/1

== system base_1fm/Robot1/DataToEtherCAT/ToActuator1/DriveEnableLogic/8_MotorAngleGuard ==
  note: This block checks whether the motor encoder gives sensible data, i.e., if the motor angle is within the expected range. The expected range is the full stroke of the output shaft plus the maximum spring deflection, transformed to motor angle space.
  To_ToActuator : Inport
  TorqueGuardMax : Inport  Port=2
  Add : Sum  Inputs=+-
  Add1 : Sum
  Bus Selector : BusSelector  OutputSignals=MotorPosition_IncEnc_rad
  Divide : Product  Inputs=*/
  Logical Operator : Logic  Operator=OR  AllPortsSameDT=off  OutDataTypeStr=boolean
  Maximum : Constant  Value=ActuatorStruct.JointAnglePositionGuardMax_rad
  Minimum : Constant  Value=ActuatorStruct.JointAnglePositionGuardMin_rad
  Relational Operator1 : RelationalOperator  Operator=<=  OutDataTypeStr=boolean  RndMeth=Nearest
  Relational Operator2 : RelationalOperator  OutDataTypeStr=boolean  RndMeth=Nearest
  SpringStiffness : Constant  Value=ActuatorStruct.SpringStiffness_Nm_rad
  TransformToMotorSpace : Gain  Gain=ActuatorStruct.gearboxRatio
  TransformToMotorSpace1 : Gain  Gain=ActuatorStruct.gearboxRatio
  Error : Outport
  wires:
  Minimum/1 -> Add/1
  Divide/1 -> Add1/2, Add/2  "MaximumSpringDeflection_rad"
  Maximum/1 -> Add1/1
  SpringStiffness/1 -> Divide/2
  TorqueGuardMax/1 -> Divide/1
  TransformToMotorSpace/1 -> Relational Operator2/2
  Add/1 -> TransformToMotorSpace1/1
  Add1/1 -> TransformToMotorSpace/1
  TransformToMotorSpace1/1 -> Relational Operator1/2
  Logical Operator/1 -> Error/1
  Relational Operator2/1 -> Logical Operator/2
  Relational Operator1/1 -> Logical Operator/1
  Bus Selector/1 -> Relational Operator1/1, Relational Operator2/1  "<MotorPosition_IncEnc_rad>"
  To_ToActuator/1 -> Bus Selector/1

== system base_1fm/Robot1/DataToEtherCAT/ToActuator1/DriveEnableLogic/CreateSingleErrorValue ==
  ErrorChecks : Inport
  Data Type Conversion1 : DataTypeConversion  OutDataTypeStr=double
  Data Type Conversion2 : DataTypeConversion  OutDataTypeStr=int32
  MATLAB Function : MATLAB Function  TreatAsAtomicUnit=on
  Select_NotUseActuator : Selector  InputPortWidth=3  IndexOptions=Index vector (dialog)  Indices=1  OutputSizes=1
  Switch : Switch  Criteria=u2 ~= 0
  Unary Minus : UnaryMinus
  Out1 : Outport
  wires:
  Unary Minus/1 -> Switch/1
  Switch/1 -> Out1/1
  ErrorChecks/1 -> Data Type Conversion1/1
  Select_NotUseActuator/1 -> Switch/2
  Data Type Conversion1/1 -> Select_NotUseActuator/1, MATLAB Function/1(errors)
  MATLAB Function/1(out) -> Data Type Conversion2/1
  Data Type Conversion2/1 -> Unary Minus/1, Switch/3

== system base_1fm/Robot1/DataToEtherCAT/ToActuator1/DriveEnableLogic/LatchRising ==
  in : Inport
  Trigger : TriggerPort  VariantControl=Variant  PortDimensions=1
  out : Outport
  wires:
  in/1 -> out/1

== system base_1fm/Robot1/DataToEtherCAT/ToActuator1/DriveEnableLogic/LatchRising1 ==
  in : Inport
  Trigger : TriggerPort  VariantControl=Variant  PortDimensions=1
  out : Outport
  wires:
  in/1 -> out/1
